simulink model "GRM_Airframe"  (R2018b)
settings: Solver=FixedStepAuto  StartTime=0.0  StopTime=T_sim  FixedStep=0.001  RelTol=1e-3
PreLoadFcn:
  | addpath('init_functions');
  | init_grm;
  | addpath('parameters');
  | para_def_grm;
values from neighbouring files (symbols this model uses):
  act_dmp = 0.6322    [para_def_grm.m]
  act_omega = 59.9250    (= 59.925)    [para_def_grm.m]
  aero = load('aero.mat')    [para_def_grm.m]
  c_be = -6.5e-3    (= -0.0065)    [init_grm.m]
  c_h_geop0 = 0    [init_grm.m]
  c_h_geope = 11e3    (= 11000)    [init_grm.m]
  c_pa0 = 101325    [init_grm.m]
  c_pe = -c_g0/c_be/sgc    (= 5.25587981272)    [init_grm.m]
  c_r0 = 6371000.79    [init_grm.m]
  c_rot = 7.292115e-5    (= 7.292115e-05)    [init_grm.m]
  c_Tmp0 = 288.15    [init_grm.m]
  d_siB_0 = 0    [para_def_grm.m]
  d_siB_max = deg2rad(1200)    [para_def_grm.m]
  d_siB_min = deg2rad(-1200)    [para_def_grm.m]
  dd_siB_max = deg2rad(50000)    [para_def_grm.m]
  dd_siB_min = deg2rad(-50000)    [para_def_grm.m]
  de_JBBB_xx = JBBB_xx_0 - JBBB_xx_e    (= 0)    [para_def_grm.m]
  de_JBBB_yy = JBBB_yy_0 - JBBB_yy_e    (= 0)    [para_def_grm.m]
  de_JBBB_zz = JBBB_zz_0 - JBBB_zz_e    (= 0)    [para_def_grm.m]
  de_mM = m_fuel_lookup(end)    [para_def_grm.m]
  F_prp = [450.52;428.7;423.25;391.61;352.34;304.35;266.17;243.26;216.92 ... (first row only)    [para_def_grm.m]
  flag_I_aero_switch = 1    [init_grm.m]
  flag_I_flat = 1    [init_grm.m]
  flag_I_gravity_switch = 1    [init_grm.m]
  flag_I_rot = 0    [init_grm.m]
  hcr = 1.4    [init_grm.m]
  J0PB_e = TBP*J0PP_e*TBP'    [para_def_grm.m]
  JMMM_0 = TBP*J0PP_0*TBP'    [para_def_grm.m]
  JMMM_e = TBP*J0PP_e*TBP'    [para_def_grm.m]
  lat_0 = 0    [init_grm.m]
  lon_0 = 0    [init_grm.m]
  m0 = mB_0    (= 3.30977)    [para_def_grm.m]
  m_fuel_lookup = [0;0.0573;0.1127;0.1667;0.2186;0.2681;0.3149;0.3588 ... (first row only)    [para_def_grm.m]
  mB_0 = 3.30977    [para_def_grm.m]
  mM_0 = 1.119    [para_def_grm.m]
  mM_e = de_mM    [para_def_grm.m]
  p0PB = [x0PB;y0PB;z0PB]    [para_def_grm.m]
  pBII_0 = TIE_0*pBEE_0    [init_grm.m]
  pMPB = [xMPB;yMPB;zMPB]    [para_def_grm.m]
  pNPB = [0;0;0]    [para_def_grm.m]
  qEG_0 = q12_from_T12(TEG)    [init_grm.m]
  qIB_0 = qumul(qIG_0,qGB_0)    [init_grm.m]
  qIE_0 = q12_from_T12(TIE_0)    [init_grm.m]
  sgc = 287.05287    [init_grm.m]
  siB_0 = 0    [para_def_grm.m]
  siB_max = deg2rad(30)    [para_def_grm.m]
  siB_min = deg2rad(-30)    [para_def_grm.m]
  t_prp1 = [0.04;0.28;0.54;1;1.48;1.99;2.51;3;3.5;3.67;3.82;4]    [para_def_grm.m]
  t_prp2 = t_prp2'    [para_def_grm.m]
  Tr3r4 = [1,1,1,1;1,1,-1,-1;-1,1,1,-1]*0.25    [para_def_grm.m]
  tRRR = 0    [para_def_grm.m]
  unc_act_bl = 0    [para_def_grm.m]
  unc_act_off = 0    [para_def_grm.m]
  unc_act_scale = 1    [para_def_grm.m]
  unc_aero_Cl_scale = 1    [para_def_grm.m]
  unc_aero_Cm_scale = 1    [para_def_grm.m]
  unc_aero_Cn_scale = 1    [para_def_grm.m]
  unc_aero_Cx_scale = 1    [para_def_grm.m]
  unc_aero_Cy_scale = 1    [para_def_grm.m]
  unc_aero_Cz_scale = 1    [para_def_grm.m]
  unc_cg_x = 0    [para_def_grm.m]
  unc_cg_y = 0    [para_def_grm.m]
  unc_cg_z = 0    [para_def_grm.m]
  unc_mB_bl = 0    [para_def_grm.m]
  unc_mB_scale = 1    [para_def_grm.m]
  unc_moi_Jxx = 0    [para_def_grm.m]
  unc_moi_Jyy = 0    [para_def_grm.m]
  unc_moi_Jzz = 0    [para_def_grm.m]
  unc_prp_scale = 1    [para_def_grm.m]
  unc_prp_x = 0    [para_def_grm.m]
  unc_prp_y = 0    [para_def_grm.m]
  unc_prp_z = 0    [para_def_grm.m]
  vBII_0 = vBEE_0 + cross(wIEI_0,pBII_0)    [init_grm.m]
  wBIB_0 = r2_from_r1_trans_q21(wBII_0,qBI_0)    [init_grm.m]
  x0PB = -0.5    [para_def_grm.m]
  xMPB = -0.9    [para_def_grm.m]
  y0PB = 0    [para_def_grm.m]
  yMPB = 0    [para_def_grm.m]
  z0PB = 0    [para_def_grm.m]
  zMPB = 0    [para_def_grm.m]
undefined symbols (not defined in the file or in its folder): c_b_WGS, c_flat, c_grav, c_rsma, d_mB_lookup, t_dmB
libraries: simulink_extras x11, simulink x3
(part 5 of 6)

== system GRM_Airframe/GRM_Airframe/motion_kinematics/calc_motion_kinematics/earth_rotation/quaternion_integration/Subsystem1 ==
  wEIE : Inport
  qIE : Inport  Port=2
  Add : Sum  Inputs=4
  Constant8 : Constant  Value=0
  Demux : Demux
  Demux1 : Demux  Outputs=3
  Gain : Gain  Gain=0.5
  Product{1..4} (4 alike) : Product
  Product5 : Product  Multiplication=Matrix(*)
  Q_1 : Constant  Value=[0 0 0 1; 0 0 1 0; 0 -1 0 0; -1 0 0 0]
  Q_2 : Constant  Value=[0 0 -1 0; 0 0 0 1; 1 0 0 0; 0 -1 0 0]
  Q_3 : Constant  Value=[0 1 0 0; -1 0 0 0; 0 0 0 1; 0 0 -1 0]
  Q_4 : Constant  Value=[1 0 0 0; 0 1 0 0; 0 0 1 0; 0 0 0 1]
  Vector Concatenate : Concatenate  NumInputs=4
  conjugate_quaternion1 : Subsystem
      mask help: conjugate a quaternion
      mask Help:
      | Name:
      | 
      |     conjugate_quaternion
      | 
      | Description:
      | 
      |     computes the conjugate quaternion
      | 
      | Inputs  [size] [data type] [unit]:
      | 
      |     quaternion q_2_1  [4] [double] [-]
      | 
      | Outputs  [size] [data type] [unit]:
      | 
      |     conjugated quaternion q_1_2  [4] [double] [-]
      mask Display: disp (' conj(q)')
  conjugate_quaternion2 : Subsystem
      mask help: conjugate a quaternion
      mask Help:
      | Name:
      | 
      |     conjugate_quaternion
      | 
      | Description:
      | 
      |     computes the conjugate quaternion
      | 
      | Inputs  [size] [data type] [unit]:
      | 
      |     quaternion q_2_1  [4] [double] [-]
      | 
      | Outputs  [size] [data type] [unit]:
      | 
      |     conjugated quaternion q_1_2  [4] [double] [-]
      mask Display: disp (' conj(q)')
  d_qIE : Outport
  wires:
  conjugate_quaternion2/1(q_conj) -> d_qIE/1  "d_qIE"
  wEIE/1 -> Demux1/1
  Demux/2 -> Product2/2  "w2"
  conjugate_quaternion1/1(q_conj) -> Product5/2  "qEI"
  Demux1/2 -> Vector Concatenate/2
  Demux/3 -> Product3/2  "w3"
  Q_4/1 -> Product4/1
  Product1/1 -> Add/1
  Gain/1 -> conjugate_quaternion2/1(q)  "d_qEI"
  Product5/1 -> Gain/1
  Q_2/1 -> Product2/1
  Vector Concatenate/1 -> Demux/1
  Demux/1 -> Product1/2  "w1"
  Demux1/1 -> Vector Concatenate/1
  Constant8/1 -> Vector Concatenate/4
  Q_1/1 -> Product1/1
  Q_3/1 -> Product3/1
  Product3/1 -> Add/3
  Product4/1 -> Add/4
  Demux/4 -> Product4/2  "w4"
  Add/1 -> Product5/1
  Product2/1 -> Add/2
  Demux1/3 -> Vector Concatenate/3
  qIE/1 -> conjugate_quaternion1/1(q)

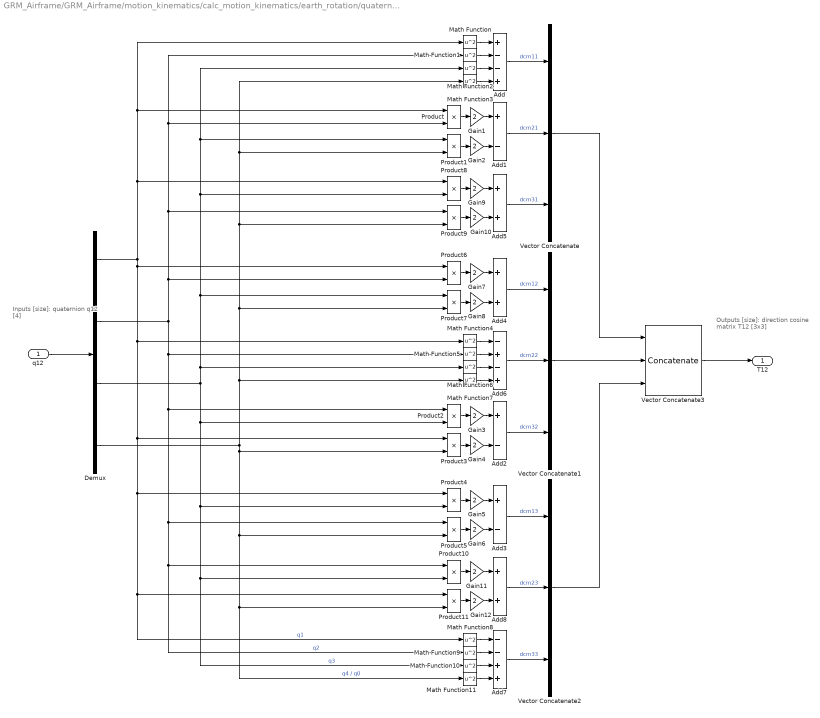
== system GRM_Airframe/GRM_Airframe/motion_kinematics/calc_motion_kinematics/earth_rotation/quaternion_integration/T12_from_q12 ==
  note: Outputs [size]:
      |
      | direction cosine matrix T12 [3x3]
  note: Inputs [size]:
      |
      | quaternion q12 [4]
  q12 : Inport  PortDimensions=4
  Add : Sum  Inputs=+--+
  Add1 : Sum  Inputs=+-
  Add2 : Sum  Inputs=+-
  Add3 : Sum  Inputs=+-
  Add4 : Sum
  Add5 : Sum
  Add6 : Sum  Inputs=-+-+
  Add7 : Sum  Inputs=--++
  Add8 : Sum
  Demux : Demux
  Gain{1..12} (12 alike) : Gain  Gain=2
  Math Function{,1..11} (12 alike) : Math  Operator=square  SaturateOnIntegerOverflow=on
  Product{,1..11} (12 alike) : Product
  Vector Concatenate : Concatenate  NumInputs=3
  Vector Concatenate1 : Concatenate  NumInputs=3
  Vector Concatenate2 : Concatenate  NumInputs=3
  Vector Concatenate3 : Concatenate  NumInputs=3  Mode=Multidimensional array  ConcatenateDimension=2
  T12 : Outport  PortDimensions=[3 3]
  wires:
  q12/1 -> Demux/1
  Demux/1 -> Product8/1, Product/1, Math Function/1, Product3/1, Product4/1, Product11/1, Math Function8/1, Math Function4/1, Product6/1  "q1"
  Demux/2 -> Product2/1, Product5/1, Product10/1, Math Function9/1, Math Function5/1, Product6/2, Product9/1, Product/2, Math Function1/1  "q2"
  Demux/3 -> Product2/2, Product4/2, Math Function10/1, Product10/2, Math Function6/1, Product7/1, Product8/2, Product1/1, Math Function2/1  "q3"
  Demux/4 -> Math Function7/1, Product7/2, Product9/2, Product1/2, Math Function3/1, Product5/2, Math Function11/1, Product11/2, Product3/2  "q4 / q0"
  Vector Concatenate3/1 -> T12/1
  Vector Concatenate/1 -> Vector Concatenate3/1
  Vector Concatenate2/1 -> Vector Concatenate3/3
  Vector Concatenate1/1 -> Vector Concatenate3/2
  Add/1 -> Vector Concatenate/1  "dcm11"
  Add1/1 -> Vector Concatenate/2  "dcm21"
  Add5/1 -> Vector Concatenate/3  "dcm31"
  Add4/1 -> Vector Concatenate1/1  "dcm12"
  Add6/1 -> Vector Concatenate1/2  "dcm22"
  Add2/1 -> Vector Concatenate1/3  "dcm32"
  Add3/1 -> Vector Concatenate2/1  "dcm13"
  Add8/1 -> Vector Concatenate2/2  "dcm23"
  Add7/1 -> Vector Concatenate2/3  "dcm33"
  Math Function/1 -> Add/1
  Math Function1/1 -> Add/2
  Math Function2/1 -> Add/3
  Math Function3/1 -> Add/4
  Product/1 -> Gain1/1
  Product1/1 -> Gain2/1
  Gain1/1 -> Add1/1
  Gain2/1 -> Add1/2
  Gain4/1 -> Add2/2
  Gain3/1 -> Add2/1
  Product3/1 -> Gain4/1
  Product2/1 -> Gain3/1
  Gain6/1 -> Add3/2
  Gain5/1 -> Add3/1
  Product5/1 -> Gain6/1
  Product4/1 -> Gain5/1
  Gain8/1 -> Add4/2
  Gain7/1 -> Add4/1
  Product7/1 -> Gain8/1
  Product6/1 -> Gain7/1
  Gain10/1 -> Add5/2
  Gain9/1 -> Add5/1
  Product9/1 -> Gain10/1
  Product8/1 -> Gain9/1
  Math Function6/1 -> Add6/3
  Math Function7/1 -> Add6/4
  Math Function5/1 -> Add6/2
  Math Function4/1 -> Add6/1
  Math Function10/1 -> Add7/3
  Math Function11/1 -> Add7/4
  Math Function9/1 -> Add7/2
  Math Function8/1 -> Add7/1
  Gain12/1 -> Add8/2
  Gain11/1 -> Add8/1
  Product11/1 -> Gain12/1
  Product10/1 -> Gain11/1

== system GRM_Airframe/GRM_Airframe/motion_kinematics/calc_motion_kinematics/earth_rotation/quaternion_integration1/Subsystem1 ==
  wGEG : Inport
  qEG : Inport  Port=2
  Add : Sum  Inputs=4
  Constant8 : Constant  Value=0
  Demux : Demux
  Demux1 : Demux  Outputs=3
  Gain : Gain  Gain=0.5
  Product{1..4} (4 alike) : Product
  Product5 : Product  Multiplication=Matrix(*)
  Q_1 : Constant  Value=[0 0 0 1; 0 0 1 0; 0 -1 0 0; -1 0 0 0]
  Q_2 : Constant  Value=[0 0 -1 0; 0 0 0 1; 1 0 0 0; 0 -1 0 0]
  Q_3 : Constant  Value=[0 1 0 0; -1 0 0 0; 0 0 0 1; 0 0 -1 0]
  Q_4 : Constant  Value=[1 0 0 0; 0 1 0 0; 0 0 1 0; 0 0 0 1]
  Vector Concatenate : Concatenate  NumInputs=4
  conjugate_quaternion1 : Subsystem
      mask help: conjugate a quaternion
      mask Help:
      | Name:
      | 
      |     conjugate_quaternion
      | 
      | Description:
      | 
      |     computes the conjugate quaternion
      | 
      | Inputs  [size] [data type] [unit]:
      | 
      |     quaternion q_2_1  [4] [double] [-]
      | 
      | Outputs  [size] [data type] [unit]:
      | 
      |     conjugated quaternion q_1_2  [4] [double] [-]
      mask Display: disp (' conj(q)')
  conjugate_quaternion2 : Subsystem
      mask help: conjugate a quaternion
      mask Help:
      | Name:
      | 
      |     conjugate_quaternion
      | 
      | Description:
      | 
      |     computes the conjugate quaternion
      | 
      | Inputs  [size] [data type] [unit]:
      | 
      |     quaternion q_2_1  [4] [double] [-]
      | 
      | Outputs  [size] [data type] [unit]:
      | 
      |     conjugated quaternion q_1_2  [4] [double] [-]
      mask Display: disp (' conj(q)')
  d_qEG : Outport
  wires:
  qEG/1 -> conjugate_quaternion1/1(q)
  Demux1/3 -> Vector Concatenate/3
  Product2/1 -> Add/2
  Add/1 -> Product5/1
  Demux/4 -> Product4/2  "w4"
  Product4/1 -> Add/4
  Product3/1 -> Add/3
  Q_3/1 -> Product3/1
  Q_1/1 -> Product1/1
  Constant8/1 -> Vector Concatenate/4
  Demux1/1 -> Vector Concatenate/1
  Demux/1 -> Product1/2  "w1"
  Vector Concatenate/1 -> Demux/1
  Q_2/1 -> Product2/1
  Product5/1 -> Gain/1
  Gain/1 -> conjugate_quaternion2/1(q)  "d_qGE"
  Product1/1 -> Add/1
  Q_4/1 -> Product4/1
  Demux/3 -> Product3/2  "w3"
  Demux1/2 -> Vector Concatenate/2
  conjugate_quaternion1/1(q_conj) -> Product5/2  "qGE"
  Demux/2 -> Product2/2  "w2"
  wGEG/1 -> Demux1/1
  conjugate_quaternion2/1(q_conj) -> d_qEG/1  "d_qEG"

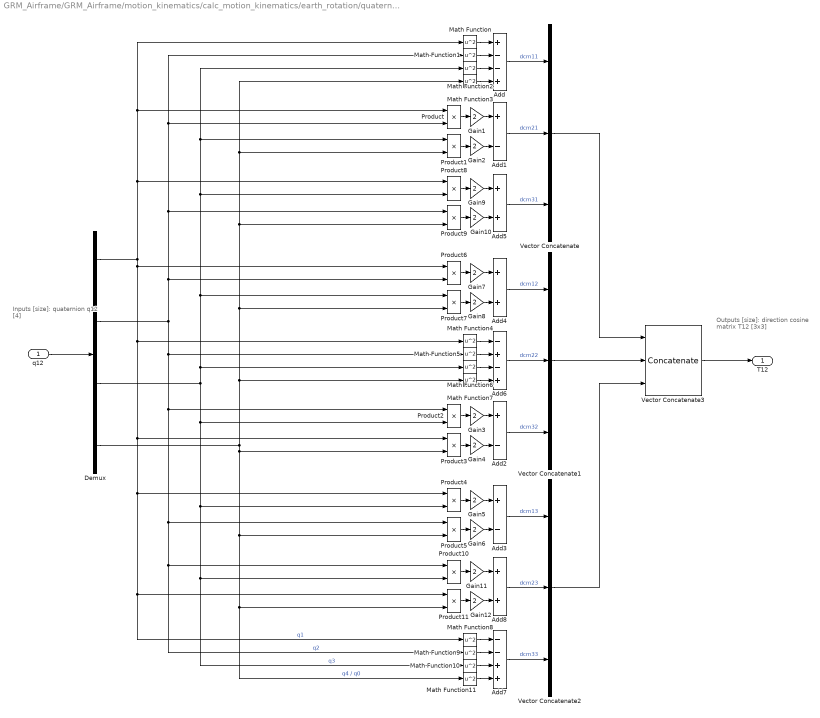
== system GRM_Airframe/GRM_Airframe/motion_kinematics/calc_motion_kinematics/earth_rotation/quaternion_integration1/T12_from_q12 ==
  note: Outputs [size]:
      |
      | direction cosine matrix T12 [3x3]
  note: Inputs [size]:
      |
      | quaternion q12 [4]
  q12 : Inport  PortDimensions=4
  Add : Sum  Inputs=+--+
  Add1 : Sum  Inputs=+-
  Add2 : Sum  Inputs=+-
  Add3 : Sum  Inputs=+-
  Add4 : Sum
  Add5 : Sum
  Add6 : Sum  Inputs=-+-+
  Add7 : Sum  Inputs=--++
  Add8 : Sum
  Demux : Demux
  Gain{1..12} (12 alike) : Gain  Gain=2
  Math Function{,1..11} (12 alike) : Math  Operator=square  SaturateOnIntegerOverflow=on
  Product{,1..11} (12 alike) : Product
  Vector Concatenate : Concatenate  NumInputs=3
  Vector Concatenate1 : Concatenate  NumInputs=3
  Vector Concatenate2 : Concatenate  NumInputs=3
  Vector Concatenate3 : Concatenate  NumInputs=3  Mode=Multidimensional array  ConcatenateDimension=2
  T12 : Outport  PortDimensions=[3 3]
  wires:
  q12/1 -> Demux/1
  Demux/1 -> Product8/1, Product/1, Math Function/1, Product3/1, Product4/1, Product11/1, Math Function8/1, Math Function4/1, Product6/1  "q1"
  Demux/2 -> Product2/1, Product5/1, Product10/1, Math Function9/1, Math Function5/1, Product6/2, Product9/1, Product/2, Math Function1/1  "q2"
  Demux/3 -> Product2/2, Product4/2, Math Function10/1, Product10/2, Math Function6/1, Product7/1, Product8/2, Product1/1, Math Function2/1  "q3"
  Demux/4 -> Math Function7/1, Product7/2, Product9/2, Product1/2, Math Function3/1, Product5/2, Math Function11/1, Product11/2, Product3/2  "q4 / q0"
  Vector Concatenate3/1 -> T12/1
  Vector Concatenate/1 -> Vector Concatenate3/1
  Vector Concatenate2/1 -> Vector Concatenate3/3
  Vector Concatenate1/1 -> Vector Concatenate3/2
  Add/1 -> Vector Concatenate/1  "dcm11"
  Add1/1 -> Vector Concatenate/2  "dcm21"
  Add5/1 -> Vector Concatenate/3  "dcm31"
  Add4/1 -> Vector Concatenate1/1  "dcm12"
  Add6/1 -> Vector Concatenate1/2  "dcm22"
  Add2/1 -> Vector Concatenate1/3  "dcm32"
  Add3/1 -> Vector Concatenate2/1  "dcm13"
  Add8/1 -> Vector Concatenate2/2  "dcm23"
  Add7/1 -> Vector Concatenate2/3  "dcm33"
  Math Function/1 -> Add/1
  Math Function1/1 -> Add/2
  Math Function2/1 -> Add/3
  Math Function3/1 -> Add/4
  Product/1 -> Gain1/1
  Product1/1 -> Gain2/1
  Gain1/1 -> Add1/1
  Gain2/1 -> Add1/2
  Gain4/1 -> Add2/2
  Gain3/1 -> Add2/1
  Product3/1 -> Gain4/1
  Product2/1 -> Gain3/1
  Gain6/1 -> Add3/2
  Gain5/1 -> Add3/1
  Product5/1 -> Gain6/1
  Product4/1 -> Gain5/1
  Gain8/1 -> Add4/2
  Gain7/1 -> Add4/1
  Product7/1 -> Gain8/1
  Product6/1 -> Gain7/1
  Gain10/1 -> Add5/2
  Gain9/1 -> Add5/1
  Product9/1 -> Gain10/1
  Product8/1 -> Gain9/1
  Math Function6/1 -> Add6/3
  Math Function7/1 -> Add6/4
  Math Function5/1 -> Add6/2
  Math Function4/1 -> Add6/1
  Math Function10/1 -> Add7/3
  Math Function11/1 -> Add7/4
  Math Function9/1 -> Add7/2
  Math Function8/1 -> Add7/1
  Gain12/1 -> Add8/2
  Gain11/1 -> Add8/1
  Product11/1 -> Gain12/1
  Product10/1 -> Gain11/1

== system GRM_Airframe/GRM_Airframe/rb_eom/calc_bus_flight_dyn_bus_entries/Subsystem2/trafo_E_to_geodetic/Geodetic_altitude ==
  pBEE : Inport
  c_rsma : Inport  Port=2
  c_flat : Inport  Port=3
  lat : Inport  Port=4
  Add : Sum
  Constant : Constant
  Gain : Gain  Gain=2
  Product : Product  Inputs=*/  SaturateOnIntegerOverflow=on  RndMeth=Zero  InputSameDT=on  OutDataTypeStr=Inherit: Same as first input
  Product1 : Product
  Product2 : Product
  Product3 : Product
  Product4 : Product  Inputs=*/  SaturateOnIntegerOverflow=on  RndMeth=Zero  InputSameDT=on  OutDataTypeStr=Inherit: Same as first input
  Product5 : Product  Inputs=3
  Selector : Selector  IndexMode=Zero-based  InputPortWidth=3  IndexOptions=Index vector (dialog)  Indices=0  OutputSizes=1
  Selector1 : Selector  IndexMode=Zero-based  InputPortWidth=3  IndexOptions=Index vector (dialog)  Indices=1  OutputSizes=1
  Sqrt : Sqrt  SaturateOnIntegerOverflow=on
  Sqrt1 : Sqrt  SaturateOnIntegerOverflow=on
  Subtract : Sum  Inputs=+-
  Subtract1 : Sum  Inputs=+-
  Sum : Sum  Inputs=+-  SaturateOnIntegerOverflow=on  InputSameDT=on  OutDataTypeStr=Inherit: Same as first input
  Trigonometric Function : Trigonometry
  cos(latGD) : Trigonometry  Operator=cos
  alt : Outport
  wires:
  lat/1 -> Trigonometric Function/1, cos(latGD)/1
  Sqrt/1 -> Product/1
  cos(latGD)/1 -> Product/2
  c_rsma/1 -> Product4/1
  Subtract/1 -> Product5/3
  Product/1 -> Sum/1
  Sum/1 -> alt/1  "alt"
  Selector/1 -> Product1/2, Product1/1
  Selector1/1 -> Product2/2, Product2/1
  Product1/1 -> Add/1
  Product2/1 -> Add/2
  Add/1 -> Sqrt/1
  pBEE/1 -> Selector1/1, Selector/1
  Product3/1 -> Subtract/2
  Gain/1 -> Subtract/1
  c_flat/1 -> Product3/1, Product3/2, Gain/1
  Sqrt1/1 -> Product4/2
  Subtract1/1 -> Sqrt1/1
  Constant/1 -> Subtract1/1
  Product5/1 -> Subtract1/2
  Trigonometric Function/1 -> Product5/2, Product5/1
  Product4/1 -> Sum/2

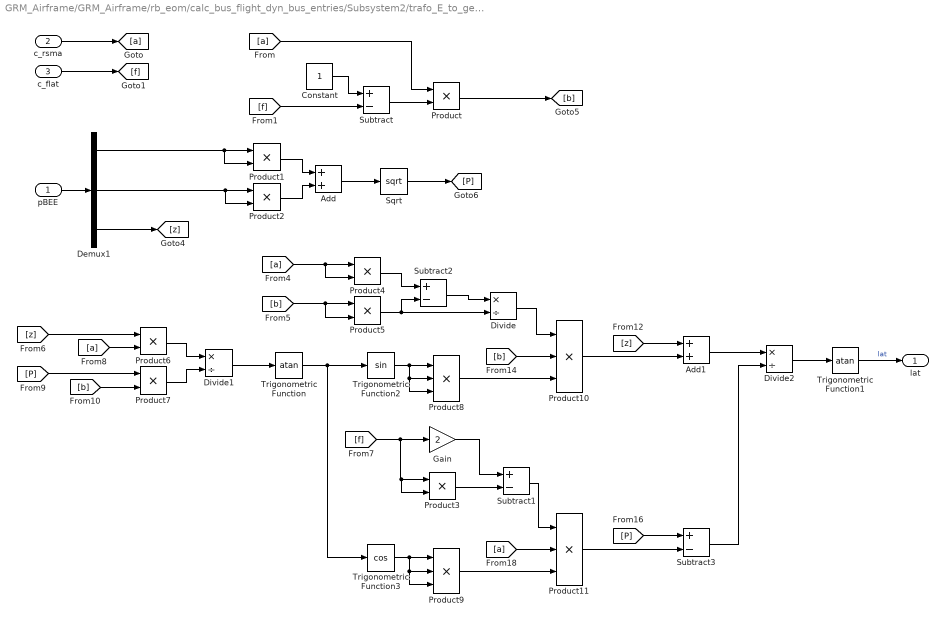
== system GRM_Airframe/GRM_Airframe/rb_eom/calc_bus_flight_dyn_bus_entries/Subsystem2/trafo_E_to_geodetic/Geodetic_latitude ==
  pBEE : Inport
  c_rsma : Inport  Port=2
  c_flat : Inport  Port=3
  Add : Sum
  Add1 : Sum
  Constant : Constant
  Demux1 : Demux  Outputs=[1;1;1]
  Divide : Product  Inputs=*/
  Divide1 : Product  Inputs=*/
  Divide2 : Product  Inputs=*/
  Gain : Gain  Gain=2
  Product{,1..7} (8 alike) : Product
  Product{8..11} (4 alike) : Product  Inputs=3
  Sqrt : Sqrt  SaturateOnIntegerOverflow=on
  Subtract{,1..3} (4 alike) : Sum  Inputs=+-
  Trigonometric Function : Trigonometry  Operator=atan
  Trigonometric Function1 : Trigonometry  Operator=atan
  Trigonometric Function2 : Trigonometry
  Trigonometric Function3 : Trigonometry  Operator=cos
  lat : Outport
  wires:
  c_flat/1 -> [f]
  c_rsma/1 -> [a]
  pBEE/1 -> Demux1/1
  Demux1/3 -> [z]
  [a] -> Product/1
  [f] -> Subtract/2
  Demux1/1 -> Product1/2, Product1/1
  Demux1/2 -> Product2/2, Product2/1
  [a] -> Product4/2, Product4/1
  [b] -> Product5/2, Product5/1
  [f] -> Product3/2, Product3/1, Gain/1
  [z] -> Product6/1
  [a] -> Product6/2
  Trigonometric Function/1 -> Trigonometric Function3/1, Trigonometric Function2/1
  [P] -> Product7/1
  [b] -> Product7/2
  [z] -> Add1/1
  [b] -> Product10/2
  [P] -> Subtract3/1
  Subtract1/1 -> Product11/1
  [a] -> Product11/2
  Trigonometric Function1/1 -> lat/1  "lat"
  Constant/1 -> Subtract/1
  Subtract/1 -> Product/2
  Product/1 -> [b]
  Product1/1 -> Add/1
  Product2/1 -> Add/2
  Add/1 -> Sqrt/1
  Sqrt/1 -> [P]
  Product3/1 -> Subtract1/2
  Gain/1 -> Subtract1/1
  Product4/1 -> Subtract2/1
  Product5/1 -> Subtract2/2, Divide/2
  Subtract2/1 -> Divide/1
  Product6/1 -> Divide1/1
  Product7/1 -> Divide1/2
  Divide1/1 -> Trigonometric Function/1
  Divide2/1 -> Trigonometric Function1/1
  Trigonometric Function2/1 -> Product8/2, Product8/3, Product8/1
  Trigonometric Function3/1 -> Product9/2, Product9/3, Product9/1
  Product8/1 -> Product10/3
  Product10/1 -> Add1/2
  Add1/1 -> Divide2/1
  Subtract3/1 -> Divide2/2
  Product11/1 -> Subtract3/2
  Product9/1 -> Product11/3
  Divide/1 -> Product10/1

== system GRM_Airframe/GRM_Airframe/rb_eom/eom_6dof/Rigid_Body_EOM_6_DOF/Integration/normalize_quaternion ==
  note: Inputs [size]:
      |
      | q [4]
  note: Outputs [size]:
      |
      | q_norm [4]
  q : Inport
  Add : Sum  Inputs=++++
  Demux : Demux  Outputs=[1;1;1;1]
  Math Function : Math  Operator=sqrt  SaturateOnIntegerOverflow=on
  Product : Product  Inputs=*/  SaturateOnIntegerOverflow=on  RndMeth=Zero  InputSameDT=on  OutDataTypeStr=Inherit: Same as first input
  Product{1..4} (4 alike) : Product  RndMeth=Zero
  q_normalized : Outport
  wires:
  Product/1 -> q_normalized/1
  q/1 -> Product/1, Demux/1
  Demux/1 -> Product1/1, Product1/2
  Demux/2 -> Product2/1, Product2/2
  Demux/3 -> Product3/1, Product3/2
  Demux/4 -> Product4/1, Product4/2
  Product4/1 -> Add/4
  Product3/1 -> Add/3
  Product2/1 -> Add/2
  Product1/1 -> Add/1
  Add/1 -> Math Function/1
  Math Function/1 -> Product/2

== system GRM_Airframe/GRM_Airframe/rb_eom/eom_6dof/Rigid_Body_EOM_6_DOF/rb_eom_6dof/calc_d_qIB ==
  note: Body-Drehraten
      | d_qBI(1) =1/2 { q4wx  - q3wy + q2wz }
      | d_qBI(2) =1/2 { q3wx + q4wy  - q1wz }
      | d_qBI(3) =1/2 {-q2wx + q1wy + q4wz }
      | d_qBI(4) =1/2 {-q1wx  - q2wy  - q3wz }
      |
      | Entspricht Zipfel (s. 372, Gl 10.11)
      | Entspricht "Representing Attitude: Euler angles, Unit Quaternions, and Rotation Vectors",
      | 	J. Diebel, Stanford University, S. 16, Gl 157 oder (159 & 151)
      |
      | d_qBI = 1/2 * [wBIB (1, 2, 3), 0] * qBI
  qIB : Inport
  wBIB : Inport  Port=2
  Add : Sum  Inputs=++++
  Constant : Constant  Value=0
  Demux : Demux  Outputs=3
  Demux1 : Demux
  Gain : Gain  Gain=0.5
  Product{2..5} (4 alike) : Product
  Product6 : Product  Multiplication=Matrix(*)
  Q_1 : Constant  Value=[0 0 0 1; 0 0 1 0; 0 -1 0 0; -1 0 0 0]
  Q_2 : Constant  Value=[0 0 -1 0; 0 0 0 1; 1 0 0 0; 0 -1 0 0]
  Q_3 : Constant  Value=[0 1 0 0; -1 0 0 0; 0 0 0 1; 0 0 -1 0]
  Q_4 : Constant  Value=[1 0 0 0; 0 1 0 0; 0 0 1 0; 0 0 0 1]
  Vector Concatenate : Concatenate  NumInputs=4
  conjugate_quaternion : Subsystem
      mask help: conjugate a quaternion
      mask Help:
      | Name:
      | 
      |     conjugate_quaternion
      | 
      | Description:
      | 
      |     computes the conjugate quaternion
      | 
      | Inputs  [size] [data type] [unit]:
      | 
      |     quaternion q_2_1  [4] [double] [-]
      | 
      | Outputs  [size] [data type] [unit]:
      | 
      |     conjugated quaternion q_1_2  [4] [double] [-]
      mask Display: disp (' conj(q)')
  conjugate_quaternion1 : Subsystem
      mask help: conjugate a quaternion
      mask Help:
      | Name:
      | 
      |     conjugate_quaternion
      | 
      | Description:
      | 
      |     computes the conjugate quaternion
      | 
      | Inputs  [size] [data type] [unit]:
      | 
      |     quaternion q_2_1  [4] [double] [-]
      | 
      | Outputs  [size] [data type] [unit]:
      | 
      |     conjugated quaternion q_1_2  [4] [double] [-]
      mask Display: disp (' conj(q)')
  d_qIB : Outport
  wires:
  Q_3/1 -> Product4/1
  Add/1 -> Product6/1  "Q(w')"
  Demux1/1 -> Product2/2  "w1"
  Product5/1 -> Add/4
  Product6/1 -> Gain/1
  Q_4/1 -> Product5/1
  Demux1/2 -> Product3/2  "w2"
  Q_1/1 -> Product2/1
  Q_2/1 -> Product3/1
  Product3/1 -> Add/2
  Demux1/3 -> Product4/2  "w3"
  Demux1/4 -> Product5/2  "w4"
  Product4/1 -> Add/3
  Product2/1 -> Add/1
  Gain/1 -> conjugate_quaternion1/1(q)  "d_qBI"
  qIB/1 -> conjugate_quaternion/1(q)
  wBIB/1 -> Demux/1
  Demux/1 -> Vector Concatenate/1
  Demux/2 -> Vector Concatenate/2
  Demux/3 -> Vector Concatenate/3
  Constant/1 -> Vector Concatenate/4
  Vector Concatenate/1 -> Demux1/1
  conjugate_quaternion/1(q_conj) -> Product6/2  "qBI"
  conjugate_quaternion1/1(q_conj) -> d_qIB/1  "d_qIB"

== system GRM_Airframe/GRM_Airframe/rb_eom/eom_6dof/Rigid_Body_EOM_6_DOF/rb_eom_6dof/cross_product ==
  note: Inputs [size]:
      |
      | r1 [3x1]
      | r2 [3x1]
  note: Outputs [size]:
      |
      | r1 x r2  [3x1]
  r1 : Inport
  r2 : Inport  Port=2
  Demux2 : Demux  Outputs=[1;1;1]
  Demux3 : Demux  Outputs=[1;1;1]
  Product{2..7} (6 alike) : Product  SaturateOnIntegerOverflow=on  RndMeth=Zero  InputSameDT=on  OutDataTypeStr=Inherit: Same as first input
  Sum : Sum  Inputs=+-  SaturateOnIntegerOverflow=on  InputSameDT=on  OutDataTypeStr=Inherit: Same as first input
  Sum1 : Sum  Inputs=+-  SaturateOnIntegerOverflow=on  InputSameDT=on  OutDataTypeStr=Inherit: Same as first input
  Sum2 : Sum  Inputs=+-  SaturateOnIntegerOverflow=on  InputSameDT=on  OutDataTypeStr=Inherit: Same as first input
  Vector Concatenate : Concatenate  NumInputs=3  Mode=Multidimensional array
  r1_x_r2 : Outport  PortDimensions=[3,1]
  wires:
  Vector Concatenate/1 -> r1_x_r2/1
  r2/1 -> Demux3/1
  r1/1 -> Demux2/1
  Sum2/1 -> Vector Concatenate/3
  Sum1/1 -> Vector Concatenate/2
  Sum/1 -> Vector Concatenate/1
  Product7/1 -> Sum2/2
  Product6/1 -> Sum2/1
  Product5/1 -> Sum1/2
  Product4/1 -> Sum1/1
  Product3/1 -> Sum/2
  Product2/1 -> Sum/1
  Demux2/1 -> Product5/1, Product6/1
  Demux3/1 -> Product4/2, Product7/2
  Demux2/3 -> Product4/1, Product3/1
  Demux3/2 -> Product3/2, Product6/2
  Demux3/3 -> Product2/2, Product5/2
  Demux2/2 -> Product7/1, Product2/1

== system GRM_Airframe/GRM_Airframe/rb_eom/eom_6dof/Rigid_Body_EOM_6_DOF/rb_eom_6dof/r2_from_r1_trans_q21 ==
  note: Inputs [size]:
      |
      | vector r1 [3]
      | quaternion q21 [4]
  note: Outputs [size]:
      |
      | vector r2 [3]
  r1 : Inport
  q21 : Inport  Port=2
  Add : Sum  Inputs=++++
  Add1 : Sum  Inputs=++++
  Constant : Constant  Value=0
  Demux : Demux  Outputs=3
  Demux1 : Demux
  Demux2 : Demux
  Math Function : Math  Operator=transpose  SaturateOnIntegerOverflow=on
  Product{,1..7} (8 alike) : Product
  Product8 : Product  Inputs=3  Multiplication=Matrix(*)
  Q_1 : Constant  Value=[0 0 0 1; 0 0 1 0; 0 -1 0 0; -1 0 0 0]
  Q_2 : Constant  Value=[0 0 -1 0; 0 0 0 1; 1 0 0 0; 0 -1 0 0]
  Q_3 : Constant  Value=[0 1 0 0; -1 0 0 0; 0 0 0 1; 0 0 -1 0]
  Q_4 : Constant  Value=[1 0 0 0; 0 1 0 0; 0 0 1 0; 0 0 0 1]
  Q~_1 : Constant  Value=[0 0 0 1; 0 0 -1 0; 0 1 0 0; -1 0 0 0]
  Q~_2 : Constant  Value=[0 0 1 0; 0 0 0 1; -1 0 0 0; 0 -1 0 0]
  Q~_3 : Constant  Value=[0 -1 0 0; 1 0 0 0; 0 0 0 1; 0 0 -1 0]
  Q~_4 : Constant  Value=[1 0 0 0; 0 1 0 0; 0 0 1 0; 0 0 0 1]
  Selector : Selector  IndexMode=Zero-based  InputPortWidth=4  IndexOptions=Index vector (dialog)  Indices=[0 1 2]  OutputSizes=1
  Vector Concatenate : Concatenate  NumInputs=4
  r2 : Outport
  wires:
  r1/1 -> Demux/1
  Demux/1 -> Vector Concatenate/1  "rx"
  Demux/2 -> Vector Concatenate/2  "ry"
  Demux/3 -> Vector Concatenate/3  "rz"
  Demux1/1 -> Product/2  "q1"
  Demux1/2 -> Product1/2  "q2"
  Demux1/3 -> Product2/2  "q3"
  Demux1/4 -> Product3/2  "q4"
  Q_1/1 -> Product/1
  Q_2/1 -> Product1/1
  Q_3/1 -> Product2/1
  Q_4/1 -> Product3/1
  Product/1 -> Add/1
  Product1/1 -> Add/2
  Product2/1 -> Add/3
  Product3/1 -> Add/4
  Add/1 -> Product8/2  "Q(q)"
  Demux2/1 -> Product4/2  "q1"
  Demux2/4 -> Product7/2  "q4"
  Q~_2/1 -> Product5/1
  Product4/1 -> Add1/1
  Product7/1 -> Add1/4
  q21/1 -> Demux2/1, Demux1/1
  Add1/1 -> Math Function/1  "Q~(q)"
  Demux2/2 -> Product5/2  "q2"
  Product5/1 -> Add1/2
  Demux2/3 -> Product6/2  "q3"
  Product6/1 -> Add1/3
  Q~_4/1 -> Product7/1
  Q~_1/1 -> Product4/1
  Q~_3/1 -> Product6/1
  Math Function/1 -> Product8/1  "Q~T(q)"
  Constant/1 -> Vector Concatenate/4
  Vector Concatenate/1 -> Product8/3
  Product8/1 -> Selector/1
  Selector/1 -> r2/1

== system GRM_Airframe/GRM_Airframe/stream_flow/calc_stream_flow/Subsystem1/AoA_Sideslip_Alphatot_Phi/norm_of_vector ==
  note: Inputs [size]:
      |
      | vector  [3]
  note: Outputs [size]:
      |
      | norm of vector [1]
  vector : Inport
  Dot Product1 : DotProduct  InputSameDT=on  OutDataTypeStr=Inherit: Inherit via internal rule
  Math Function1 : Math  Operator=sqrt  SaturateOnIntegerOverflow=on
  norm_of_vector : Outport
  wires:
  Dot Product1/1 -> Math Function1/1
  Math Function1/1 -> norm_of_vector/1
  vector/1 -> Dot Product1/2, Dot Product1/1

== system GRM_Airframe/GRM_Airframe/weight_and_balance/moi/moi_coordinate_transformation/3_rot_mat/1. Rotation x-Achse ==
  alpha1 : Inport
  Constant : Constant
  Constant{1..2,7..8} (4 alike) : Constant  Value=0
  Gain : Gain  Gain=-1
  Matrix Concatenate : Concatenate  NumInputs=3  Mode=Multidimensional array  ConcatenateDimension=2
  Mux : Mux  Inputs=3
  Mux1 : Mux  Inputs=3
  Mux2 : Mux  Inputs=3
  Trigonometric Function : Trigonometry  Operator=cos
  Trigonometric Function1 : Trigonometry
  Trigonometric Function2 : Trigonometry
  Trigonometric Function3 : Trigonometry  Operator=cos
  1Rot_Matrix_x : Outport
  wires:
  Matrix Concatenate/1 -> 1Rot_Matrix_x/1
  Mux2/1 -> Matrix Concatenate/3
  Mux1/1 -> Matrix Concatenate/2
  Mux/1 -> Matrix Concatenate/1
  Trigonometric Function3/1 -> Mux2/3
  Trigonometric Function1/1 -> Mux2/2
  Constant7/1 -> Mux2/1
  Trigonometric Function2/1 -> Gain/1
  Trigonometric Function/1 -> Mux1/2
  Constant8/1 -> Mux1/1
  Constant2/1 -> Mux/3
  Constant1/1 -> Mux/2
  Constant/1 -> Mux/1
  alpha1/1 -> Trigonometric Function3/1, Trigonometric Function1/1, Trigonometric Function/1, Trigonometric Function2/1
  Gain/1 -> Mux1/3

== system GRM_Airframe/GRM_Airframe/weight_and_balance/moi/moi_coordinate_transformation/3_rot_mat/1. Rotation y-Achse ==
  alpha1 : Inport
  Constant{,2,7..8} (4 alike) : Constant  Value=0
  Constant1 : Constant
  Gain1 : Gain  Gain=-1
  Matrix Concatenate : Concatenate  NumInputs=3  Mode=Multidimensional array  ConcatenateDimension=2
  Mux : Mux  Inputs=3
  Mux1 : Mux  Inputs=3
  Mux2 : Mux  Inputs=3
  Trigonometric Function : Trigonometry  Operator=cos
  Trigonometric Function1 : Trigonometry
  Trigonometric Function2 : Trigonometry
  Trigonometric Function3 : Trigonometry  Operator=cos
  1Rot_Matrix_y : Outport
  wires:
  Matrix Concatenate/1 -> 1Rot_Matrix_y/1
  Constant7/1 -> Mux2/2
  Trigonometric Function2/1 -> Mux/3
  Trigonometric Function/1 -> Mux/1
  Constant8/1 -> Mux/2
  alpha1/1 -> Trigonometric Function/1, Trigonometric Function2/1, Trigonometric Function3/1, Trigonometric Function1/1
  Constant/1 -> Mux1/1
  Constant1/1 -> Mux1/2
  Constant2/1 -> Mux1/3
  Trigonometric Function1/1 -> Gain1/1
  Trigonometric Function3/1 -> Mux2/3
  Mux/1 -> Matrix Concatenate/1
  Mux1/1 -> Matrix Concatenate/2
  Mux2/1 -> Matrix Concatenate/3
  Gain1/1 -> Mux2/1

== system GRM_Airframe/GRM_Airframe/weight_and_balance/moi/moi_coordinate_transformation/3_rot_mat/1. Rotation z-Achse ==
  alpha1 : Inport
  Constant{4,7..8,10} (4 alike) : Constant  Value=0
  Constant11 : Constant
  Gain : Gain  Gain=-1
  Matrix Concatenate : Concatenate  NumInputs=3  Mode=Multidimensional array  ConcatenateDimension=2
  Mux : Mux  Inputs=3
  Mux1 : Mux  Inputs=3
  Mux2 : Mux  Inputs=3
  Trigonometric Function : Trigonometry  Operator=cos
  Trigonometric Function1 : Trigonometry
  Trigonometric Function3 : Trigonometry  Operator=cos
  Trigonometric Function4 : Trigonometry
  1Rot_Matrix_z : Outport
  wires:
  alpha1/1 -> Trigonometric Function1/1, Trigonometric Function/1, Trigonometric Function4/1, Trigonometric Function3/1
  Matrix Concatenate/1 -> 1Rot_Matrix_z/1
  Constant8/1 -> Mux/3
  Trigonometric Function4/1 -> Gain/1
  Trigonometric Function3/1 -> Mux/1
  Constant11/1 -> Mux2/3
  Constant10/1 -> Mux2/2
  Constant4/1 -> Mux2/1
  Constant7/1 -> Mux1/3
  Trigonometric Function1/1 -> Mux1/1
  Mux2/1 -> Matrix Concatenate/3
  Mux1/1 -> Matrix Concatenate/2
  Mux/1 -> Matrix Concatenate/1
  Trigonometric Function/1 -> Mux1/2
  Gain/1 -> Mux/2

== system GRM_Airframe/GRM_Airframe/weight_and_balance/moi/moi_coordinate_transformation/3_rot_mat/2. Rotation x-Achse ==
  alpha2 : Inport
  Constant : Constant
  Constant{1..2,7..8} (4 alike) : Constant  Value=0
  Gain : Gain  Gain=-1
  Matrix Concatenate : Concatenate  NumInputs=3  Mode=Multidimensional array  ConcatenateDimension=2
  Mux : Mux  Inputs=3
  Mux1 : Mux  Inputs=3
  Mux2 : Mux  Inputs=3
  Trigonometric Function : Trigonometry  Operator=cos
  Trigonometric Function1 : Trigonometry
  Trigonometric Function2 : Trigonometry
  Trigonometric Function3 : Trigonometry  Operator=cos
  2Rot_Matrix_x : Outport
  wires:
  Matrix Concatenate/1 -> 2Rot_Matrix_x/1
  Mux2/1 -> Matrix Concatenate/3
  Mux1/1 -> Matrix Concatenate/2
  Mux/1 -> Matrix Concatenate/1
  Trigonometric Function3/1 -> Mux2/3
  Trigonometric Function1/1 -> Mux2/2
  Constant7/1 -> Mux2/1
  Trigonometric Function2/1 -> Gain/1
  Trigonometric Function/1 -> Mux1/2
  Constant8/1 -> Mux1/1
  Constant2/1 -> Mux/3
  Constant1/1 -> Mux/2
  Constant/1 -> Mux/1
  alpha2/1 -> Trigonometric Function3/1, Trigonometric Function1/1, Trigonometric Function/1, Trigonometric Function2/1
  Gain/1 -> Mux1/3

== system GRM_Airframe/GRM_Airframe/weight_and_balance/moi/moi_coordinate_transformation/3_rot_mat/2. Rotation y-Achse ==
  alpha2 : Inport
  Constant{,2,7..8} (4 alike) : Constant  Value=0
  Constant1 : Constant
  Gain1 : Gain  Gain=-1
  Matrix Concatenate : Concatenate  NumInputs=3  Mode=Multidimensional array  ConcatenateDimension=2
  Mux : Mux  Inputs=3
  Mux1 : Mux  Inputs=3
  Mux2 : Mux  Inputs=3
  Trigonometric Function : Trigonometry  Operator=cos
  Trigonometric Function1 : Trigonometry
  Trigonometric Function2 : Trigonometry
  Trigonometric Function3 : Trigonometry  Operator=cos
  2Rot_Matrix_y : Outport
  wires:
  Matrix Concatenate/1 -> 2Rot_Matrix_y/1
  Constant7/1 -> Mux2/2
  Trigonometric Function2/1 -> Mux/3
  Trigonometric Function/1 -> Mux/1
  Constant8/1 -> Mux/2
  alpha2/1 -> Trigonometric Function/1, Trigonometric Function2/1, Trigonometric Function3/1, Trigonometric Function1/1
  Constant/1 -> Mux1/1
  Constant1/1 -> Mux1/2
  Constant2/1 -> Mux1/3
  Trigonometric Function1/1 -> Gain1/1
  Trigonometric Function3/1 -> Mux2/3
  Mux/1 -> Matrix Concatenate/1
  Mux1/1 -> Matrix Concatenate/2
  Mux2/1 -> Matrix Concatenate/3
  Gain1/1 -> Mux2/1

== system GRM_Airframe/GRM_Airframe/weight_and_balance/moi/moi_coordinate_transformation/3_rot_mat/2. Rotation z-Achse ==
  alpha2 : Inport
  Constant{4,7..8,10} (4 alike) : Constant  Value=0
  Constant11 : Constant
  Gain : Gain  Gain=-1
  Matrix Concatenate : Concatenate  NumInputs=3  Mode=Multidimensional array  ConcatenateDimension=2
  Mux : Mux  Inputs=3
  Mux1 : Mux  Inputs=3
  Mux2 : Mux  Inputs=3
  Trigonometric Function : Trigonometry  Operator=cos
  Trigonometric Function1 : Trigonometry
  Trigonometric Function3 : Trigonometry  Operator=cos
  Trigonometric Function4 : Trigonometry
  2Rot_Matrix_z : Outport
  wires:
  alpha2/1 -> Trigonometric Function1/1, Trigonometric Function/1, Trigonometric Function4/1, Trigonometric Function3/1
  Matrix Concatenate/1 -> 2Rot_Matrix_z/1
  Constant8/1 -> Mux/3
  Trigonometric Function4/1 -> Gain/1
  Trigonometric Function3/1 -> Mux/1
  Constant11/1 -> Mux2/3
  Constant10/1 -> Mux2/2
  Constant4/1 -> Mux2/1
  Constant7/1 -> Mux1/3
  Trigonometric Function1/1 -> Mux1/1
  Mux2/1 -> Matrix Concatenate/3
  Mux1/1 -> Matrix Concatenate/2
  Mux/1 -> Matrix Concatenate/1
  Trigonometric Function/1 -> Mux1/2
  Gain/1 -> Mux/2

== system GRM_Airframe/GRM_Airframe/weight_and_balance/moi/moi_coordinate_transformation/3_rot_mat/3. Rotation x-Achse ==
  alpha3 : Inport
  Constant : Constant
  Constant{1..2,7..8} (4 alike) : Constant  Value=0
  Gain : Gain  Gain=-1
  Matrix Concatenate : Concatenate  NumInputs=3  Mode=Multidimensional array  ConcatenateDimension=2
  Mux : Mux  Inputs=3
  Mux1 : Mux  Inputs=3
  Mux2 : Mux  Inputs=3
  Trigonometric Function : Trigonometry  Operator=cos
  Trigonometric Function1 : Trigonometry
  Trigonometric Function2 : Trigonometry
  Trigonometric Function3 : Trigonometry  Operator=cos
  3Rot_Matrix_x : Outport
  wires:
  Matrix Concatenate/1 -> 3Rot_Matrix_x/1
  Mux2/1 -> Matrix Concatenate/3
  Mux1/1 -> Matrix Concatenate/2
  Mux/1 -> Matrix Concatenate/1
  Trigonometric Function3/1 -> Mux2/3
  Trigonometric Function1/1 -> Mux2/2
  Constant7/1 -> Mux2/1
  Trigonometric Function2/1 -> Gain/1
  Trigonometric Function/1 -> Mux1/2
  Constant8/1 -> Mux1/1
  Constant2/1 -> Mux/3
  Constant1/1 -> Mux/2
  Constant/1 -> Mux/1
  alpha3/1 -> Trigonometric Function3/1, Trigonometric Function1/1, Trigonometric Function/1, Trigonometric Function2/1
  Gain/1 -> Mux1/3

== system GRM_Airframe/GRM_Airframe/weight_and_balance/moi/moi_coordinate_transformation/3_rot_mat/3. Rotation y-Achse ==
  alpha3 : Inport
  Constant{,2,7..8} (4 alike) : Constant  Value=0
  Constant1 : Constant
  Gain1 : Gain  Gain=-1
  Matrix Concatenate : Concatenate  NumInputs=3  Mode=Multidimensional array  ConcatenateDimension=2
  Mux : Mux  Inputs=3
  Mux1 : Mux  Inputs=3
  Mux2 : Mux  Inputs=3
  Trigonometric Function : Trigonometry  Operator=cos
  Trigonometric Function1 : Trigonometry
  Trigonometric Function2 : Trigonometry
  Trigonometric Function3 : Trigonometry  Operator=cos
  3Rot_Matrix_y : Outport
  wires:
  Matrix Concatenate/1 -> 3Rot_Matrix_y/1
  Constant7/1 -> Mux2/2
  Trigonometric Function2/1 -> Mux/3
  Trigonometric Function/1 -> Mux/1
  Constant8/1 -> Mux/2
  alpha3/1 -> Trigonometric Function/1, Trigonometric Function2/1, Trigonometric Function3/1, Trigonometric Function1/1
  Constant/1 -> Mux1/1
  Constant1/1 -> Mux1/2
  Constant2/1 -> Mux1/3
  Trigonometric Function1/1 -> Gain1/1
  Trigonometric Function3/1 -> Mux2/3
  Mux/1 -> Matrix Concatenate/1
  Mux1/1 -> Matrix Concatenate/2
  Mux2/1 -> Matrix Concatenate/3
  Gain1/1 -> Mux2/1

== system GRM_Airframe/GRM_Airframe/weight_and_balance/moi/moi_coordinate_transformation/3_rot_mat/3. Rotation z-Achse ==
  alpha3 : Inport
  Constant{4,7..8,10} (4 alike) : Constant  Value=0
  Constant11 : Constant
  Gain : Gain  Gain=-1
  Matrix Concatenate : Concatenate  NumInputs=3  Mode=Multidimensional array  ConcatenateDimension=2
  Mux : Mux  Inputs=3
  Mux1 : Mux  Inputs=3
  Mux2 : Mux  Inputs=3
  Trigonometric Function : Trigonometry  Operator=cos
  Trigonometric Function1 : Trigonometry
  Trigonometric Function3 : Trigonometry  Operator=cos
  Trigonometric Function4 : Trigonometry
  3Rot_Matrix_z : Outport
  wires:
  alpha3/1 -> Trigonometric Function1/1, Trigonometric Function/1, Trigonometric Function4/1, Trigonometric Function3/1
  Matrix Concatenate/1 -> 3Rot_Matrix_z/1
  Constant8/1 -> Mux/3
  Trigonometric Function4/1 -> Gain/1
  Trigonometric Function3/1 -> Mux/1
  Constant11/1 -> Mux2/3
  Constant10/1 -> Mux2/2
  Constant4/1 -> Mux2/1
  Constant7/1 -> Mux1/3
  Trigonometric Function1/1 -> Mux1/1
  Mux2/1 -> Matrix Concatenate/3
  Mux1/1 -> Matrix Concatenate/2
  Mux/1 -> Matrix Concatenate/1
  Trigonometric Function/1 -> Mux1/2
  Gain/1 -> Mux/2

== system GRM_Airframe/GRM_Airframe/aerodynamics/aerodynamic_via_lookup/calc_aero_for_mom/launch_rail/initial_altitude/trafo_E_to_geodetic ==
  note: Inputs [size]:
      |
      | position_E [3]
  note: Outputs [size]:
      |
      | geodetic longitude [1]
      | geodetic latitude [1]
      | geodetic altitude [1]
  pBEE : Inport
  Geodetic_altitude : Subsystem
  Geodetic_latitude : Subsystem
  Selector1 : Selector  IndexMode=Zero-based  InputPortWidth=3  IndexOptions=Index vector (dialog)  Indices=1  OutputSizes=1
  Selector2 : Selector  IndexMode=Zero-based  InputPortWidth=3  IndexOptions=Index vector (dialog)  Indices=0  OutputSizes=1
  Trigonometric Function1 : Trigonometry  Operator=atan2
  c_flat : Constant  Value=c_flat
  c_rsma : Constant  Value=c_rsma
  lon : Outport
  lat : Outport  Port=2
  alt : Outport  Port=3
  wires:
  pBEE/1 -> Geodetic_altitude/1(pBEE), Geodetic_latitude/1(pBEE), Selector2/1, Selector1/1  "pBEE"
  Trigonometric Function1/1 -> lon/1  "lon"
  Geodetic_altitude/1(alt) -> alt/1
  Geodetic_latitude/1(lat) -> lat/1, Geodetic_altitude/4(lat)
  Selector2/1 -> Trigonometric Function1/2  "pBEE_x"
  Selector1/1 -> Trigonometric Function1/1  "pBEE_y"
  c_rsma/1 -> Geodetic_altitude/2(c_rsma), Geodetic_latitude/2(c_rsma)  "c_rsma"
  c_flat/1 -> Geodetic_latitude/3(c_flat), Geodetic_altitude/3(c_flat)  "c_flat"

== system GRM_Airframe/GRM_Airframe/aerodynamics/aerodynamic_via_lookup/calc_aero_for_mom/launch_rail1/initial_altitude/trafo_E_to_geodetic ==
  note: Inputs [size]:
      |
      | position_E [3]
  note: Outputs [size]:
      |
      | geodetic longitude [1]
      | geodetic latitude [1]
      | geodetic altitude [1]
  pBEE : Inport
  Geodetic_altitude : Subsystem
  Geodetic_latitude : Subsystem
  Selector1 : Selector  IndexMode=Zero-based  InputPortWidth=3  IndexOptions=Index vector (dialog)  Indices=1  OutputSizes=1
  Selector2 : Selector  IndexMode=Zero-based  InputPortWidth=3  IndexOptions=Index vector (dialog)  Indices=0  OutputSizes=1
  Trigonometric Function1 : Trigonometry  Operator=atan2
  c_flat : Constant  Value=c_flat
  c_rsma : Constant  Value=c_rsma
  lon : Outport
  lat : Outport  Port=2
  alt : Outport  Port=3
  wires:
  pBEE/1 -> Geodetic_altitude/1(pBEE), Geodetic_latitude/1(pBEE), Selector2/1, Selector1/1  "pBEE"
  Trigonometric Function1/1 -> lon/1  "lon"
  Geodetic_altitude/1(alt) -> alt/1
  Geodetic_latitude/1(lat) -> lat/1, Geodetic_altitude/4(lat)
  Selector2/1 -> Trigonometric Function1/2  "pBEE_x"
  Selector1/1 -> Trigonometric Function1/1  "pBEE_y"
  c_rsma/1 -> Geodetic_altitude/2(c_rsma), Geodetic_latitude/2(c_rsma)  "c_rsma"
  c_flat/1 -> Geodetic_latitude/3(c_flat), Geodetic_altitude/3(c_flat)  "c_flat"

== system GRM_Airframe/GRM_Airframe/motion_kinematics/calc_motion_kinematics/earth_rotation/quaternion_integration/Subsystem1/conjugate_quaternion1 ==
  note: Inputs [size]:
      |
      | q [4]
  note: Outputs [size]:
      |
      | q_conj [4]
  q : Inport
  Demux : Demux  Outputs=[3;1]
  Gain1 : Gain  Gain=-1
  Vector Concatenate : Concatenate
  q_conj : Outport
  wires:
  q/1 -> Demux/1
  Vector Concatenate/1 -> q_conj/1
  Demux/1 -> Gain1/1
  Gain1/1 -> Vector Concatenate/1
  Demux/2 -> Vector Concatenate/2

== system GRM_Airframe/GRM_Airframe/motion_kinematics/calc_motion_kinematics/earth_rotation/quaternion_integration/Subsystem1/conjugate_quaternion2 ==
  note: Inputs [size]:
      |
      | q [4]
  note: Outputs [size]:
      |
      | q_conj [4]
  q : Inport
  Demux : Demux  Outputs=[3;1]
  Gain1 : Gain  Gain=-1
  Vector Concatenate : Concatenate
  q_conj : Outport
  wires:
  q/1 -> Demux/1
  Vector Concatenate/1 -> q_conj/1
  Demux/1 -> Gain1/1
  Gain1/1 -> Vector Concatenate/1
  Demux/2 -> Vector Concatenate/2

== system GRM_Airframe/GRM_Airframe/motion_kinematics/calc_motion_kinematics/earth_rotation/quaternion_integration1/Subsystem1/conjugate_quaternion1 ==
  note: Inputs [size]:
      |
      | q [4]
  note: Outputs [size]:
      |
      | q_conj [4]
  q : Inport
  Demux : Demux  Outputs=[3;1]
  Gain1 : Gain  Gain=-1
  Vector Concatenate : Concatenate
  q_conj : Outport
  wires:
  q/1 -> Demux/1
  Vector Concatenate/1 -> q_conj/1
  Demux/1 -> Gain1/1
  Gain1/1 -> Vector Concatenate/1
  Demux/2 -> Vector Concatenate/2

== system GRM_Airframe/GRM_Airframe/motion_kinematics/calc_motion_kinematics/earth_rotation/quaternion_integration1/Subsystem1/conjugate_quaternion2 ==
  note: Inputs [size]:
      |
      | q [4]
  note: Outputs [size]:
      |
      | q_conj [4]
  q : Inport
  Demux : Demux  Outputs=[3;1]
  Gain1 : Gain  Gain=-1
  Vector Concatenate : Concatenate
  q_conj : Outport
  wires:
  q/1 -> Demux/1
  Vector Concatenate/1 -> q_conj/1
  Demux/1 -> Gain1/1
  Gain1/1 -> Vector Concatenate/1
  Demux/2 -> Vector Concatenate/2

== system GRM_Airframe/GRM_Airframe/rb_eom/eom_6dof/Rigid_Body_EOM_6_DOF/rb_eom_6dof/calc_d_qIB/conjugate_quaternion ==
  note: Inputs [size]:
      |
      | q [4]
  note: Outputs [size]:
      |
      | q_conj [4]
  q : Inport
  Demux : Demux  Outputs=[3;1]
  Gain1 : Gain  Gain=-1
  Vector Concatenate : Concatenate
  q_conj : Outport
  wires:
  q/1 -> Demux/1
  Vector Concatenate/1 -> q_conj/1
  Demux/1 -> Gain1/1
  Gain1/1 -> Vector Concatenate/1
  Demux/2 -> Vector Concatenate/2

== system GRM_Airframe/GRM_Airframe/rb_eom/eom_6dof/Rigid_Body_EOM_6_DOF/rb_eom_6dof/calc_d_qIB/conjugate_quaternion1 ==
  note: Inputs [size]:
      |
      | q [4]
  note: Outputs [size]:
      |
      | q_conj [4]
  q : Inport
  Demux : Demux  Outputs=[3;1]
  Gain1 : Gain  Gain=-1
  Vector Concatenate : Concatenate
  q_conj : Outport
  wires:
  q/1 -> Demux/1
  Vector Concatenate/1 -> q_conj/1
  Demux/1 -> Gain1/1
  Gain1/1 -> Vector Concatenate/1
  Demux/2 -> Vector Concatenate/2

== system GRM_Airframe/GRM_Airframe/aerodynamics/aerodynamic_via_lookup/calc_aero_for_mom/launch_rail/initial_altitude/trafo_E_to_geodetic/Geodetic_altitude ==
  pBEE : Inport
  c_rsma : Inport  Port=2
  c_flat : Inport  Port=3
  lat : Inport  Port=4
  Add : Sum
  Constant : Constant
  Gain : Gain  Gain=2
  Product : Product  Inputs=*/  SaturateOnIntegerOverflow=on  RndMeth=Zero  InputSameDT=on  OutDataTypeStr=Inherit: Same as first input
  Product1 : Product
  Product2 : Product
  Product3 : Product
  Product4 : Product  Inputs=*/  SaturateOnIntegerOverflow=on  RndMeth=Zero  InputSameDT=on  OutDataTypeStr=Inherit: Same as first input
  Product5 : Product  Inputs=3
  Selector : Selector  IndexMode=Zero-based  InputPortWidth=3  IndexOptions=Index vector (dialog)  Indices=0  OutputSizes=1
  Selector1 : Selector  IndexMode=Zero-based  InputPortWidth=3  IndexOptions=Index vector (dialog)  Indices=1  OutputSizes=1
  Sqrt : Sqrt  SaturateOnIntegerOverflow=on
  Sqrt1 : Sqrt  SaturateOnIntegerOverflow=on
  Subtract : Sum  Inputs=+-
  Subtract1 : Sum  Inputs=+-
  Sum : Sum  Inputs=+-  SaturateOnIntegerOverflow=on  InputSameDT=on  OutDataTypeStr=Inherit: Same as first input
  Trigonometric Function : Trigonometry
  cos(latGD) : Trigonometry  Operator=cos
  alt : Outport
  wires:
  lat/1 -> Trigonometric Function/1, cos(latGD)/1
  Sqrt/1 -> Product/1
  cos(latGD)/1 -> Product/2
  c_rsma/1 -> Product4/1
  Subtract/1 -> Product5/3
  Product/1 -> Sum/1
  Sum/1 -> alt/1  "alt"
  Selector/1 -> Product1/2, Product1/1
  Selector1/1 -> Product2/2, Product2/1
  Product1/1 -> Add/1
  Product2/1 -> Add/2
  Add/1 -> Sqrt/1
  pBEE/1 -> Selector1/1, Selector/1
  Product3/1 -> Subtract/2
  Gain/1 -> Subtract/1
  c_flat/1 -> Product3/1, Product3/2, Gain/1
  Sqrt1/1 -> Product4/2
  Subtract1/1 -> Sqrt1/1
  Constant/1 -> Subtract1/1
  Product5/1 -> Subtract1/2
  Trigonometric Function/1 -> Product5/2, Product5/1
  Product4/1 -> Sum/2

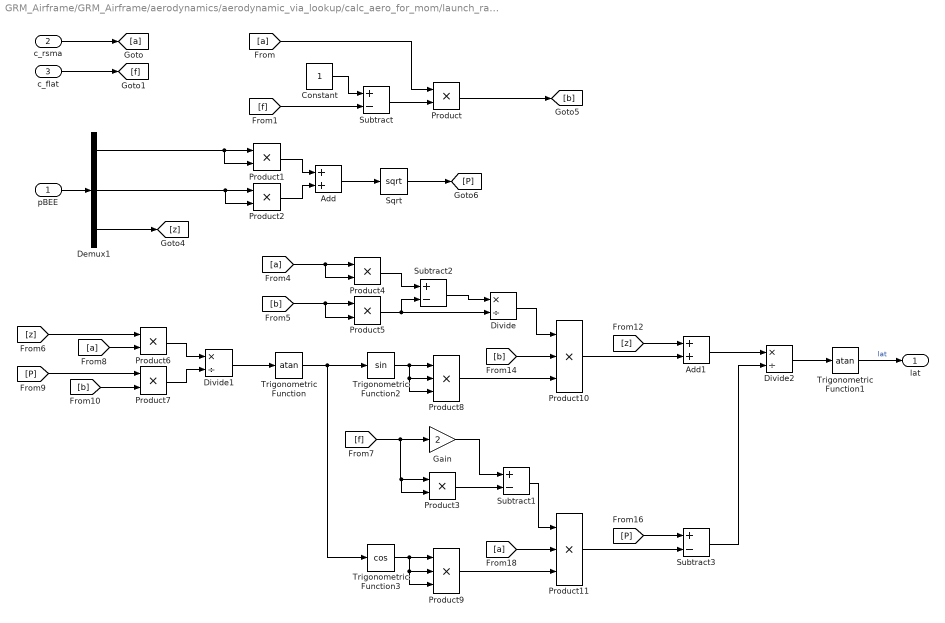
== system GRM_Airframe/GRM_Airframe/aerodynamics/aerodynamic_via_lookup/calc_aero_for_mom/launch_rail/initial_altitude/trafo_E_to_geodetic/Geodetic_latitude ==
  pBEE : Inport
  c_rsma : Inport  Port=2
  c_flat : Inport  Port=3
  Add : Sum
  Add1 : Sum
  Constant : Constant
  Demux1 : Demux  Outputs=[1;1;1]
  Divide : Product  Inputs=*/
  Divide1 : Product  Inputs=*/
  Divide2 : Product  Inputs=*/
  Gain : Gain  Gain=2
  Product{,1..7} (8 alike) : Product
  Product{8..11} (4 alike) : Product  Inputs=3
  Sqrt : Sqrt  SaturateOnIntegerOverflow=on
  Subtract{,1..3} (4 alike) : Sum  Inputs=+-
  Trigonometric Function : Trigonometry  Operator=atan
  Trigonometric Function1 : Trigonometry  Operator=atan
  Trigonometric Function2 : Trigonometry
  Trigonometric Function3 : Trigonometry  Operator=cos
  lat : Outport
  wires:
  c_flat/1 -> [f]
  c_rsma/1 -> [a]
  pBEE/1 -> Demux1/1
  Demux1/3 -> [z]
  [a] -> Product/1
  [f] -> Subtract/2
  Demux1/1 -> Product1/2, Product1/1
  Demux1/2 -> Product2/2, Product2/1
  [a] -> Product4/2, Product4/1
  [b] -> Product5/2, Product5/1
  [f] -> Product3/2, Product3/1, Gain/1
  [z] -> Product6/1
  [a] -> Product6/2
  Trigonometric Function/1 -> Trigonometric Function3/1, Trigonometric Function2/1
  [P] -> Product7/1
  [b] -> Product7/2
  [z] -> Add1/1
  [b] -> Product10/2
  [P] -> Subtract3/1
  Subtract1/1 -> Product11/1
  [a] -> Product11/2
  Trigonometric Function1/1 -> lat/1  "lat"
  Constant/1 -> Subtract/1
  Subtract/1 -> Product/2
  Product/1 -> [b]
  Product1/1 -> Add/1
  Product2/1 -> Add/2
  Add/1 -> Sqrt/1
  Sqrt/1 -> [P]
  Product3/1 -> Subtract1/2
  Gain/1 -> Subtract1/1
  Product4/1 -> Subtract2/1
  Product5/1 -> Subtract2/2, Divide/2
  Subtract2/1 -> Divide/1
  Product6/1 -> Divide1/1
  Product7/1 -> Divide1/2
  Divide1/1 -> Trigonometric Function/1
  Divide2/1 -> Trigonometric Function1/1
  Trigonometric Function2/1 -> Product8/2, Product8/3, Product8/1
  Trigonometric Function3/1 -> Product9/2, Product9/3, Product9/1
  Product8/1 -> Product10/3
  Product10/1 -> Add1/2
  Add1/1 -> Divide2/1
  Subtract3/1 -> Divide2/2
  Product11/1 -> Subtract3/2
  Product9/1 -> Product11/3
  Divide/1 -> Product10/1

== system GRM_Airframe/GRM_Airframe/aerodynamics/aerodynamic_via_lookup/calc_aero_for_mom/launch_rail1/initial_altitude/trafo_E_to_geodetic/Geodetic_altitude ==
  pBEE : Inport
  c_rsma : Inport  Port=2
  c_flat : Inport  Port=3
  lat : Inport  Port=4
  Add : Sum
  Constant : Constant
  Gain : Gain  Gain=2
  Product : Product  Inputs=*/  SaturateOnIntegerOverflow=on  RndMeth=Zero  InputSameDT=on  OutDataTypeStr=Inherit: Same as first input
  Product1 : Product
  Product2 : Product
  Product3 : Product
  Product4 : Product  Inputs=*/  SaturateOnIntegerOverflow=on  RndMeth=Zero  InputSameDT=on  OutDataTypeStr=Inherit: Same as first input
  Product5 : Product  Inputs=3
  Selector : Selector  IndexMode=Zero-based  InputPortWidth=3  IndexOptions=Index vector (dialog)  Indices=0  OutputSizes=1
  Selector1 : Selector  IndexMode=Zero-based  InputPortWidth=3  IndexOptions=Index vector (dialog)  Indices=1  OutputSizes=1
  Sqrt : Sqrt  SaturateOnIntegerOverflow=on
  Sqrt1 : Sqrt  SaturateOnIntegerOverflow=on
  Subtract : Sum  Inputs=+-
  Subtract1 : Sum  Inputs=+-
  Sum : Sum  Inputs=+-  SaturateOnIntegerOverflow=on  InputSameDT=on  OutDataTypeStr=Inherit: Same as first input
  Trigonometric Function : Trigonometry
  cos(latGD) : Trigonometry  Operator=cos
  alt : Outport
  wires:
  lat/1 -> Trigonometric Function/1, cos(latGD)/1
  Sqrt/1 -> Product/1
  cos(latGD)/1 -> Product/2
  c_rsma/1 -> Product4/1
  Subtract/1 -> Product5/3
  Product/1 -> Sum/1
  Sum/1 -> alt/1  "alt"
  Selector/1 -> Product1/2, Product1/1
  Selector1/1 -> Product2/2, Product2/1
  Product1/1 -> Add/1
  Product2/1 -> Add/2
  Add/1 -> Sqrt/1
  pBEE/1 -> Selector1/1, Selector/1
  Product3/1 -> Subtract/2
  Gain/1 -> Subtract/1
  c_flat/1 -> Product3/1, Product3/2, Gain/1
  Sqrt1/1 -> Product4/2
  Subtract1/1 -> Sqrt1/1
  Constant/1 -> Subtract1/1
  Product5/1 -> Subtract1/2
  Trigonometric Function/1 -> Product5/2, Product5/1
  Product4/1 -> Sum/2
